simulink model "MIMO_36Channel_Model"  (R2024b)
settings: Solver=VariableStepAuto  StartTime=0.0  StopTime=10.0  RelTol=1e-3
settings Model: Creator=kevin  LastModifiedBy=kevin

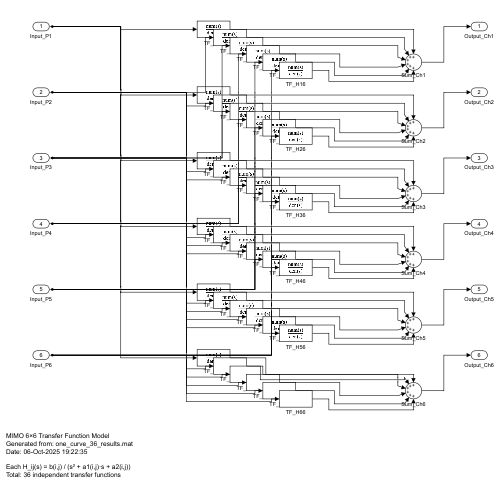
[thumbnail: Simulink's stored preview of the top-level diagram]
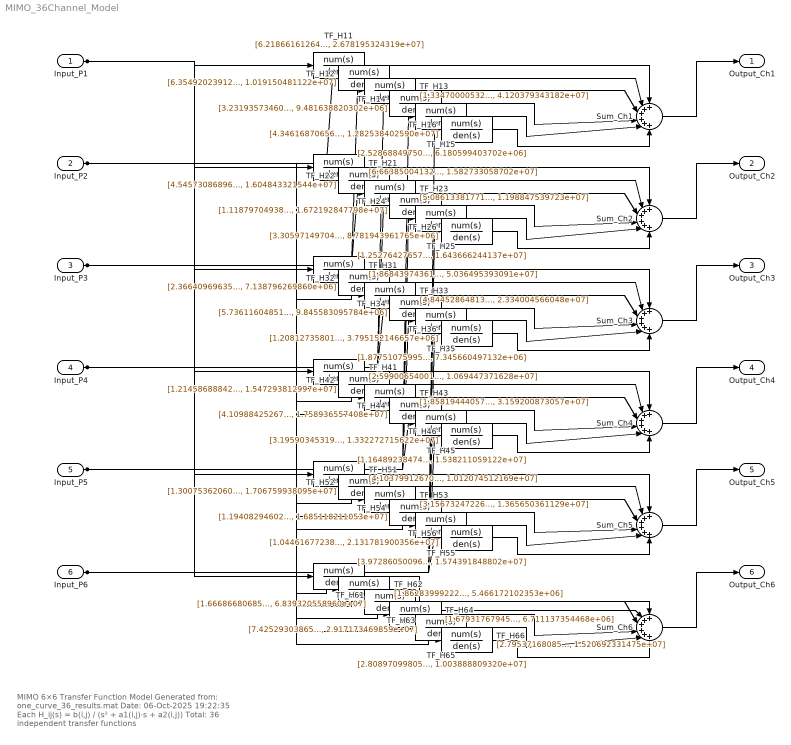
== system MIMO_36Channel_Model ==
  note: MIMO 6×6 Transfer Function Model
      | Generated from: one_curve_36_results.mat
      | Date: 06-Oct-2025 19:22:35
      |
      | Each H_ij(s) = b(i,j) / (s² + a1(i,j)·s + a2(i,j))
      | Total: 36 independent transfer functions
  Input_P1 : Inport
  Input_P2 : Inport  Port=2
  Input_P3 : Inport  Port=3
  Input_P4 : Inport  Port=4
  Input_P5 : Inport  Port=5
  Input_P6 : Inport  Port=6
  Sum_Ch{1..6} (6 alike) : Sum  Inputs=++++++
  TF_H11 : TransferFcn  Numerator=[6.218661612646e+06]  Denominator=[1, 1.338651505722e+04, 2.678195324319e+07]
  TF_H12 : TransferFcn  Numerator=[6.354920239120e+04]  Denominator=[1, 1.662975234098e+03, 1.019150481122e+07]
  TF_H13 : TransferFcn  Numerator=[1.334700005324e+06]  Denominator=[1, 1.275258720887e+04, 4.120379343182e+07]
  TF_H14 : TransferFcn  Numerator=[3.231935734603e+05]  Denominator=[1, 7.852044258687e+03, 9.481638820302e+06]
  TF_H15 : TransferFcn  Numerator=[2.528688497505e+05]  Denominator=[1, 5.879364609866e+03, 6.180599403702e+06]
  TF_H16 : TransferFcn  Numerator=[4.346168706564e+05]  Denominator=[1, 3.929701077901e+03, 1.282538402590e+07]
  TF_H21 : TransferFcn  Numerator=[6.663850041322e+04]  Denominator=[1, 1.462325866359e+03, 1.582733058702e+07]
  TF_H22 : TransferFcn  Numerator=[4.545730868967e+06]  Denominator=[1, 1.062107240072e+04, 1.604843321544e+07]
  TF_H23 : TransferFcn  Numerator=[5.086133817713e+05]  Denominator=[1, 8.903580767443e+03, 1.198847539723e+07]
  TF_H24 : TransferFcn  Numerator=[1.118797049382e+06]  Denominator=[1, 1.187110606946e+04, 1.672192847798e+07]
  TF_H25 : TransferFcn  Numerator=[1.252764276578e+06]  Denominator=[1, 1.157065537065e+04, 1.643666244137e+07]
  TF_H26 : TransferFcn  Numerator=[3.305971497046e+05]  Denominator=[1, 7.320553639319e+03, 8.781943961765e+06]
  TF_H31 : TransferFcn  Numerator=[1.868439743615e+06]  Denominator=[1, 2.001759478912e+04, 5.036495393091e+07]
  TF_H32 : TransferFcn  Numerator=[2.366409696351e+05]  Denominator=[1, 5.555556272703e+03, 7.138796269860e+06]
  TF_H33 : TransferFcn  Numerator=[4.844528648136e+06]  Denominator=[1, 9.879529061686e+03, 2.334004566048e+07]
  TF_H34 : TransferFcn  Numerator=[5.736116048513e+04]  Denominator=[1, 1.969312774925e+03, 9.845583095784e+06]
  TF_H35 : TransferFcn  Numerator=[1.877510759958e+05]  Denominator=[1, 5.415723666298e+03, 7.345660497132e+06]
  TF_H36 : TransferFcn  Numerator=[1.208127358015e+05]  Denominator=[1, 1.223159436233e+03, 3.795152146657e+06]
  TF_H41 : TransferFcn  Numerator=[2.599006540014e+05]  Denominator=[1, 7.067011596941e+03, 1.069447371628e+07]
  TF_H42 : TransferFcn  Numerator=[1.214586888427e+06]  Denominator=[1, 1.068737062822e+04, 1.547293812997e+07]
  TF_H43 : TransferFcn  Numerator=[1.858194440575e+05]  Denominator=[1, 3.263628987101e+03, 3.159200873057e+07]
  TF_H44 : TransferFcn  Numerator=[4.109884252673e+06]  Denominator=[1, 1.197023152306e+04, 1.758936557408e+07]
  TF_H45 : TransferFcn  Numerator=[1.164892384743e+06]  Denominator=[1, 1.147497418550e+04, 1.538211059122e+07]
  TF_H46 : TransferFcn  Numerator=[3.195903453190e+05]  Denominator=[1, 8.115803419255e+03, 1.332272715622e+07]
  TF_H51 : TransferFcn  Numerator=[4.103799126701e+05]  Denominator=[1, 8.911718423988e+03, 1.012074512169e+07]
  TF_H52 : TransferFcn  Numerator=[1.300753620602e+06]  Denominator=[1, 1.129883111396e+04, 1.706759938095e+07]
  TF_H53 : TransferFcn  Numerator=[3.156732472269e+05]  Denominator=[1, 7.923123695230e+03, 1.365650361129e+07]
  TF_H54 : TransferFcn  Numerator=[1.194082946029e+06]  Denominator=[1, 1.165860639982e+04, 1.685118211053e+07]
  TF_H55 : TransferFcn  Numerator=[3.972860500964e+06]  Denominator=[1, 1.114673978611e+04, 1.574391848802e+07]
  TF_H56 : TransferFcn  Numerator=[1.044616772387e+05]  Denominator=[1, 1.795313113853e+03, 2.131781900356e+07]
  TF_H61 : TransferFcn  Numerator=[1.666866806856e+06]  Denominator=[1, 2.393920383335e+04, 6.839320558960e+07]
  TF_H62 : TransferFcn  Numerator=[1.862839992228e+05]  Denominator=[1, 4.466579568847e+03, 5.466172102353e+06]
  TF_H63 : TransferFcn  Numerator=[7.425293038651e+05]  Denominator=[1, 9.585044147566e+03, 2.917173469859e+07]
  TF_H64 : TransferFcn  Numerator=[1.679317679458e+05]  Denominator=[1, 5.027625797834e+03, 6.711137354468e+06]
  TF_H65 : TransferFcn  Numerator=[2.808970998056e+04]  Denominator=[1, 4.816641149236e+02, 1.003888809320e+07]
  TF_H66 : TransferFcn  Numerator=[2.795371680855e+06]  Denominator=[1, 6.650113581422e+03, 1.520692331475e+07]
  Output_Ch1 : Outport
  Output_Ch2 : Outport  Port=2
  Output_Ch3 : Outport  Port=3
  Output_Ch4 : Outport  Port=4
  Output_Ch5 : Outport  Port=5
  Output_Ch6 : Outport  Port=6
  wires:
  Sum_Ch1/1 -> Output_Ch1/1
  Input_P1/1 -> TF_H11/1, TF_H21/1, TF_H31/1, TF_H41/1, TF_H51/1, TF_H61/1
  TF_H11/1 -> Sum_Ch1/1
  Input_P2/1 -> TF_H12/1, TF_H22/1, TF_H32/1, TF_H42/1, TF_H52/1, TF_H62/1
  TF_H12/1 -> Sum_Ch1/2
  Input_P3/1 -> TF_H13/1, TF_H23/1, TF_H33/1, TF_H43/1, TF_H53/1, TF_H63/1
  TF_H13/1 -> Sum_Ch1/3
  Input_P4/1 -> TF_H14/1, TF_H24/1, TF_H34/1, TF_H44/1, TF_H54/1, TF_H64/1
  TF_H14/1 -> Sum_Ch1/4
  Input_P5/1 -> TF_H15/1, TF_H25/1, TF_H35/1, TF_H45/1, TF_H55/1, TF_H65/1
  TF_H15/1 -> Sum_Ch1/5
  Input_P6/1 -> TF_H16/1, TF_H26/1, TF_H36/1, TF_H46/1, TF_H56/1, TF_H66/1
  TF_H16/1 -> Sum_Ch1/6
  Sum_Ch2/1 -> Output_Ch2/1
  TF_H21/1 -> Sum_Ch2/1
  TF_H22/1 -> Sum_Ch2/2
  TF_H23/1 -> Sum_Ch2/3
  TF_H24/1 -> Sum_Ch2/4
  TF_H25/1 -> Sum_Ch2/5
  TF_H26/1 -> Sum_Ch2/6
  Sum_Ch3/1 -> Output_Ch3/1
  TF_H31/1 -> Sum_Ch3/1
  TF_H32/1 -> Sum_Ch3/2
  TF_H33/1 -> Sum_Ch3/3
  TF_H34/1 -> Sum_Ch3/4
  TF_H35/1 -> Sum_Ch3/5
  TF_H36/1 -> Sum_Ch3/6
  Sum_Ch4/1 -> Output_Ch4/1
  TF_H41/1 -> Sum_Ch4/1
  TF_H42/1 -> Sum_Ch4/2
  TF_H43/1 -> Sum_Ch4/3
  TF_H44/1 -> Sum_Ch4/4
  TF_H45/1 -> Sum_Ch4/5
  TF_H46/1 -> Sum_Ch4/6
  Sum_Ch5/1 -> Output_Ch5/1
  TF_H51/1 -> Sum_Ch5/1
  TF_H52/1 -> Sum_Ch5/2
  TF_H53/1 -> Sum_Ch5/3
  TF_H54/1 -> Sum_Ch5/4
  TF_H55/1 -> Sum_Ch5/5
  TF_H56/1 -> Sum_Ch5/6
  Sum_Ch6/1 -> Output_Ch6/1
  TF_H61/1 -> Sum_Ch6/1
  TF_H62/1 -> Sum_Ch6/2
  TF_H63/1 -> Sum_Ch6/3
  TF_H64/1 -> Sum_Ch6/4
  TF_H65/1 -> Sum_Ch6/5
  TF_H66/1 -> Sum_Ch6/6
